simulink model "walkingRobotInvKin"  (R2017a)
settings: Solver=ode15s  StartTime=0.0  StopTime=10  MaxStep=1e-2  EnableMultiTasking=on
undefined symbols (not defined in the file): ankle_servo_kd, ankle_servo_ki, ankle_servo_kp, curveData, deriv_filter_coeff, foot_height_offset, foot_x, foot_y, foot_z, gaitPeriod, height_plane, initAnglesR, joint_stiffness, lower_leg_length, plane_x, plane_y, stepHeight, stepLength, torso_offset_x, torso_offset_z, torso_x, torso_y, torso_z, upper_leg_length, X, Y, Z
libraries: sm_lib x53, walkingRobotUtils x20, Contact_Forces_Lib x16, nesl_utility x8, simulink x2
(part 3 of 3)

== matlab function walkingRobotInvKin/Robot/Leg IK R ==
  data: x input; t1 output; y input; t2 output; foot_height_offset parameter; upper_leg_length parameter; lower_leg_length parameter
function [t1,t2] = invKin2D(x,y, foot_height_offset, upper_leg_length, lower_leg_length)

    % Call symbolic generated function
    theta = legInvKin(upper_leg_length/100,lower_leg_length/100,... 
                      -x,y-foot_height_offset/100);
    
    % Address multiple outputs
    if size(theta,1) == 2
       if theta(1,2) < 0
          t1 = theta(2,1);
          t2 = theta(2,2);
       else
          t1 = theta(1,1);
          t2 = theta(1,2);
       end
    else
        t1 = theta(1);
        t2 = theta(2);
    end
    
end

== matlab function walkingRobotInvKin/Robot/Leg IK L ==
  data: x input; t1 output; y input; t2 output; foot_height_offset parameter; upper_leg_length parameter; lower_leg_length parameter
function [t1,t2] = invKin2D(x,y, foot_height_offset, upper_leg_length, lower_leg_length)

    % Call symbolic generated function
    theta = legInvKin(upper_leg_length/100,lower_leg_length/100,... 
                      -x,y-foot_height_offset/100);
    
    % Address multiple outputs
    if size(theta,1) == 2
       if theta(1,2) < 0
          t1 = theta(2,1);
          t2 = theta(2,2);
       else
          t1 = theta(1,1);
          t2 = theta(1,2);
       end
    else
        t1 = theta(1);
        t2 = theta(2);
    end
    
end

== matlab function walkingRobotInvKin/Robot/Evaluate Foot Trajectory R ==
  settings: sampleTime=0.01
  data: t input; x output; y output; stepLength parameter; stepHeight parameter; gaitPeriod parameter
function [x,y] = footTraj(t, stepLength, stepHeight, gaitPeriod)
    
    [x,y] = evalFootGait(t,stepLength,stepHeight,gaitPeriod);

end

== matlab function walkingRobotInvKin/Robot/Leg IK R1 ==
  data: x input; t1 output; y input; t2 output; foot_height_offset parameter; upper_leg_length parameter; lower_leg_length parameter
function [t1,t2] = invKin2D(x,y, foot_height_offset, upper_leg_length, lower_leg_length)

    % Call symbolic generated function
    theta = legInvKin(upper_leg_length/100,lower_leg_length/100,... 
                      -x,y-foot_height_offset/100);
    
    % Address multiple outputs
    if size(theta,1) == 2
       if theta(1,2) < 0
          t1 = theta(2,1);
          t2 = theta(2,2);
       else
          t1 = theta(1,1);
          t2 = theta(1,2);
       end
    else
        t1 = theta(1);
        t2 = theta(2);
    end
    
end

== matlab function walkingRobotInvKin/Robot/Evaluate Foot Trajectory R1 ==
  settings: sampleTime=0.01
  data: t input; x output; y output; stepLength parameter; stepHeight parameter; gaitPeriod parameter
function [x,y] = footTraj(t, stepLength, stepHeight, gaitPeriod)
    
    [x,y] = evalFootGait(t,stepLength,stepHeight,gaitPeriod);

end

== matlab function walkingRobotInvKin/Robot/Leg IK L1 ==
  data: x input; t1 output; y input; t2 output; foot_height_offset parameter; upper_leg_length parameter; lower_leg_length parameter
function [t1,t2] = invKin2D(x,y, foot_height_offset, upper_leg_length, lower_leg_length)

    % Call symbolic generated function
    theta = legInvKin(upper_leg_length/100,lower_leg_length/100,... 
                      -x,y-foot_height_offset/100);
    
    % Address multiple outputs
    if size(theta,1) == 2
       if theta(1,2) < 0
          t1 = theta(2,1);
          t2 = theta(2,2);
       else
          t1 = theta(1,1);
          t2 = theta(1,2);
       end
    else
        t1 = theta(1);
        t2 = theta(2);
    end
    
end

== matlab function walkingRobotInvKin/Robot/Evaluate Foot Trajectory L1 ==
  data: t input; x output; y output; stepLength parameter; stepHeight parameter; gaitPeriod parameter
function [x,y] = footTraj(t, stepLength, stepHeight, gaitPeriod)
    
    [x,y] = evalFootGait(t,stepLength,stepHeight,gaitPeriod);

end
